simulink model "Ultrafiltration"  (R2025b)
settings: Solver=FixedStepAuto  StartTime=0.0  StopTime=1440  FixedStep=1  RelTol=1e-3
InitFcn:
  | initUF
  | tic;
StartFcn:
  | disp("Start...")
StopFcn:
  | disp("Stop...")
  | fprintf("SimTime: %.02f min", toc/60)
values from neighbouring files (symbols this model uses):
  BW_Max_Time = 90    [initUF.m]
  BW_Max_Vol_gal = 5000    [initUF.m]
  CEB_Max_Time = 1000    [initUF.m]
  CEB_Max_Vol_gal = 5000    [initUF.m]
  CIP_Max_Time = 15000    [initUF.m]
undefined symbols (not defined in the file or in its folder): LUT
libraries: simulink x30
(part 1 of 5)
PostSaveFcn:
  | disp("PostSave...")
PauseFcn:
  | disp("Pause...")
settings Model: Creator=joshl  LastModifiedBy=joshl
settings RTWCC: GPUComputeCapability=3.5

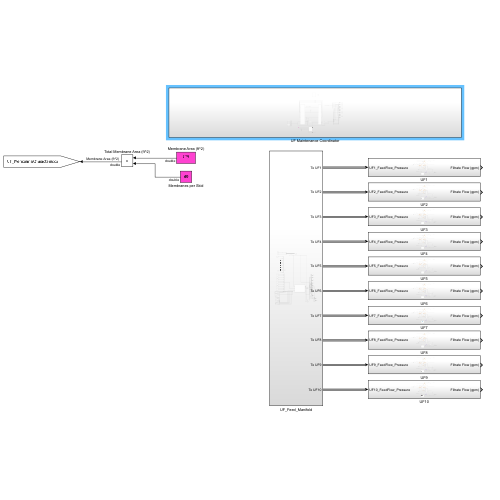
[thumbnail: Simulink's stored preview of the top-level diagram]
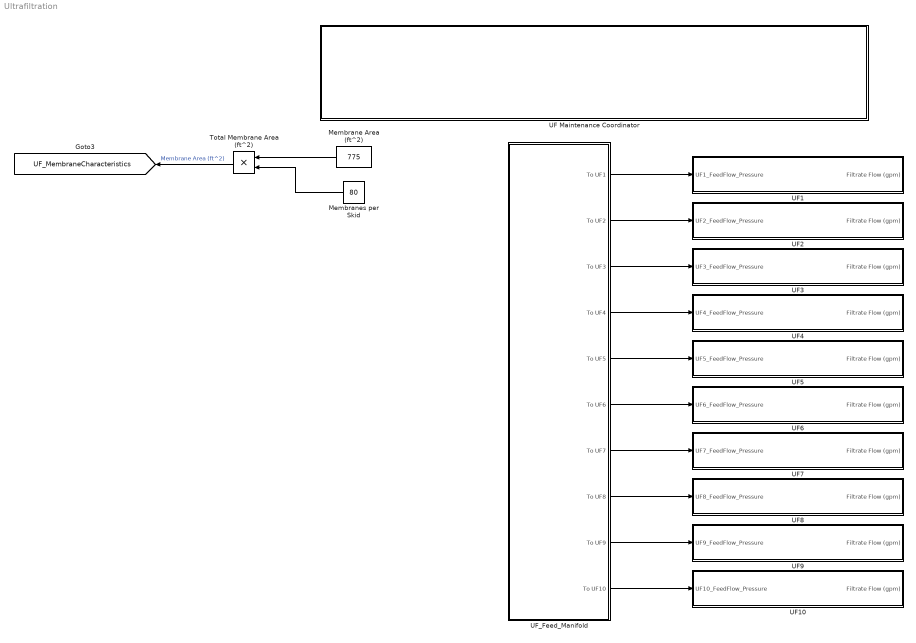
== system Ultrafiltration ==
  Membrane Area (ft^2) : Constant  Value=775
  Membranes per Skid : Constant  Value=80
  Total Membrane Area (ft^2) : Product
  UF Maintenance Coordinator : Subsystem
  UF1 : Subsystem
  UF10 : Subsystem
  UF2 : Subsystem
  UF3 : Subsystem
  UF4 : Subsystem
  UF5 : Subsystem
  UF6 : Subsystem
  UF7 : Subsystem
  UF8 : Subsystem
  UF9 : Subsystem
  UF_Feed_Manifold : Subsystem
  tag scope: UF_MembraneCharacteristics=global
  wires:
  UF_Feed_Manifold/1(To UF1) -> UF1/1(UF1_FeedFlow_Pressure)
  UF_Feed_Manifold/2(To UF2) -> UF2/1(UF2_FeedFlow_Pressure)
  Membrane Area (ft^2)/1 -> Total Membrane Area (ft^2)/1
  Membranes per Skid/1 -> Total Membrane Area (ft^2)/2
  Total Membrane Area (ft^2)/1 -> [UF_MembraneCharacteristics]  "Membrane Area (ft^2)"
  UF_Feed_Manifold/3(To UF3) -> UF3/1(UF3_FeedFlow_Pressure)
  UF_Feed_Manifold/4(To UF4) -> UF4/1(UF4_FeedFlow_Pressure)
  UF_Feed_Manifold/5(To UF5) -> UF5/1(UF5_FeedFlow_Pressure)
  UF_Feed_Manifold/6(To UF6) -> UF6/1(UF6_FeedFlow_Pressure)
  UF_Feed_Manifold/7(To UF7) -> UF7/1(UF7_FeedFlow_Pressure)
  UF_Feed_Manifold/8(To UF8) -> UF8/1(UF8_FeedFlow_Pressure)
  UF_Feed_Manifold/9(To UF9) -> UF9/1(UF9_FeedFlow_Pressure)
  UF_Feed_Manifold/10(To UF10) -> UF10/1(UF10_FeedFlow_Pressure)

== system Ultrafiltration/UF Maintenance Coordinator ==
  Bus Creator{,1..9} (10 alike) : BusCreator  Inputs=2
  Constant : Constant  Value=10000
  Demux : Demux  Outputs=10
  Demux1 : Demux  Outputs=10
  Maint Queue Vector2 : Mux  Inputs=10
  Memory{,1..3} (4 alike) : Memory
  Rate Limiter : RateLimiter  RisingSlewLimit=10000/108  FallingSlewLimit=-10000/37  SampleTimeMode=inherited
  Sample_Stateflows : Stateflow chart  Commented=on  TreatAsAtomicUnit=on
  Scope : Scope  NumInputPorts=2
      settings: DataLoggingVariableName=ScopeData2
  Scope1 : Scope  NumInputPorts=3
      settings: ActiveDisplayYMinimum=-0.12499999999999997  ActiveDisplayYMaximum=1.125
  Scope{2..5} (4 alike) : Scope
      Scope2 settings: ActiveDisplayYMinimum=-1  ActiveDisplayYMaximum=1  DataLoggingVariableName=ScopeData14
      Scope3 settings: ActiveDisplayYMinimum=-1  ActiveDisplayYMaximum=1  DataLoggingVariableName=ScopeData15
      Scope4 settings: ActiveDisplayYMinimum=-129.2228584451866  ActiveDisplayYMaximum=1163.0057260066797  DataLoggingVariableName=ScopeData16
      Scope5 settings: ActiveDisplayYMinimum=-1.2345292012789748  ActiveDisplayYMaximum=1.3904707987210259  DataLoggingVariableName=ScopeData17
  Scope6 : Scope  NumInputPorts=2
      settings: ActiveDisplayYMinimum=-0.12499999999999997  ActiveDisplayYMaximum=1.125  DataLoggingVariableName=ScopeData18
  UF Flow Maximum (gpm) : Constant  Value=1640
  UF_Dispatcher : MATLAB Function  TreatAsAtomicUnit=on
  UF_FIFO_Coordinator : MATLAB Function  Priority=100  TreatAsAtomicUnit=on  SystemSampleTime=1
  UF_State_Tracker : MATLAB Function  TreatAsAtomicUnit=on  SystemSampleTime=1
  arhive : Subsystem
  tag scope: UF10_State=global, UF1_State=global, UF2_State=global, UF3_State=global, UF4_State=global, UF5_State=global, UF6_State=global, UF7_State=global, UF8_State=global, UF9_State=global, UF_Flow_Assignment=global, UF_Operations_States_vector=global
  wires:
  UF_State_Tracker/3(operations_states) -> Scope5/1, [UF_Operations_States_vector], UF_FIFO_Coordinator/3(operating_states)
  UF_State_Tracker/1(in_startup_queue) -> Scope3/1, UF_FIFO_Coordinator/1(startup_req)
  UF_State_Tracker/2(in_maint_queue) -> Scope2/1, UF_FIFO_Coordinator/2(maint_req)
  UF_State_Tracker/4(maintenance_completion_indicators) -> Scope6/1, Scope1/3, [UF_Maintenance_Completion_Signals]  "Maintenance Completion"
  UF_FIFO_Coordinator/1(startup_cmd) -> Memory/1
  UF_FIFO_Coordinator/2(maint_cmd) -> Memory1/1
  Memory/1 -> UF_State_Tracker/1(startup_cmd)
  Memory1/1 -> UF_State_Tracker/2(maint_cmd)
  UF_FIFO_Coordinator/3(shutdown_cmd) -> Memory2/1
  Memory2/1 -> UF_State_Tracker/3(shutdown_cmd)
  UF_Dispatcher/1(flows) -> UF_FIFO_Coordinator/4(flows), Scope4/1, Memory3/1
  Rate Limiter/1 -> Scope/1, UF_Dispatcher/2(flow_actual)  "Plant Feed Actual"
  Memory3/1 -> UF_Dispatcher/4(prev_flows)
  UF Flow Maximum (gpm)/1 -> UF_Dispatcher/1(max_flow_per_unit)
  [UF2_Maintenance_Request] -> Maint Queue Vector2/2
  [UF3_Maintenance_Request] -> Maint Queue Vector2/3
  [UF7_Maintenance_Request] -> Maint Queue Vector2/7
  [UF8_Maintenance_Request] -> Maint Queue Vector2/8
  [UF5_Maintenance_Request] -> Maint Queue Vector2/5
  [UF6_Maintenance_Request] -> Maint Queue Vector2/6
  [UF10_Maintenance_Request] -> Maint Queue Vector2/10
  [UF9_Maintenance_Request] -> Maint Queue Vector2/9
  [UF4_Maintenance_Request] -> Maint Queue Vector2/4
  [UF1_Maintenance_Request] -> Maint Queue Vector2/1
  [UF_Maintenance_Completion_Signals] -> Demux/1
  Maint Queue Vector2/1 -> Scope6/2, UF_State_Tracker/4(maint_req)
  Constant/1 -> Rate Limiter/1, Scope/2, UF_Dispatcher/3(flow_setpoint)
  Demux/1 -> Bus Creator/1  "UF1_MaintenanceCompletion_signal"
  Bus Creator/1 -> [UF1_State]
  Demux/2 -> Bus Creator1/1  "UF2_MaintenanceCompletion_signal"
  Demux/3 -> Bus Creator2/1  "UF3_MaintenanceCompletion_signal"
  Demux/4 -> Bus Creator3/1  "UF4_MaintenanceCompletion_signal"
  Demux/5 -> Bus Creator4/1  "UF5_MaintenanceCompletion_signal"
  Bus Creator1/1 -> [UF2_State]
  Demux/6 -> Bus Creator5/1  "UF6_MaintenanceCompletion_signal"
  Bus Creator3/1 -> [UF4_State]
  Bus Creator2/1 -> [UF3_State]
  Bus Creator5/1 -> [UF6_State]
  Bus Creator4/1 -> [UF5_State]
  Bus Creator7/1 -> [UF8_State]
  Bus Creator6/1 -> [UF7_State]
  Bus Creator9/1 -> [UF10_State]
  Bus Creator8/1 -> [UF9_State]
  Demux/7 -> Bus Creator6/1  "UF7_MaintenanceCompletion_signal"
  Demux/8 -> Bus Creator7/1  "UF8_MaintenanceCompletion_signal"
  Demux/9 -> Bus Creator8/1  "UF9_MaintenanceCompletion_signal"
  Demux/10 -> Bus Creator9/1  "UF10_MaintenanceCompletion_signal"
  Demux1/2 -> Bus Creator1/2  "UF2_OperationsState_signal"
  Demux1/7 -> Bus Creator6/2  "UF7_OperationsState_signal"
  Demux1/10 -> Bus Creator9/2  "UF10_OperationsState_signal"
  Demux1/1 -> Bus Creator/2  "UF1_OperationsState_signal"
  Demux1/8 -> Bus Creator7/2  "UF8_OperationsState_signal"
  Demux1/4 -> Bus Creator3/2  "UF4_OperationsState_signal"
  Demux1/9 -> Bus Creator8/2  "UF9_OperationsState_signal"
  Demux1/3 -> Bus Creator2/2  "UF3_OperationsState_signal"
  [UF_Operations_States_vector] -> Scope1/1, Demux1/1  "OperationsStates"
  Demux1/5 -> Bus Creator4/2  "UF5_OperationsState_signal"
  Demux1/6 -> Bus Creator5/2  "UF6_OperationsState_signal"
  UF_FIFO_Coordinator/4(assigned_flows) -> Scope1/2, [UF_Flow_Assignment]  "Flows"

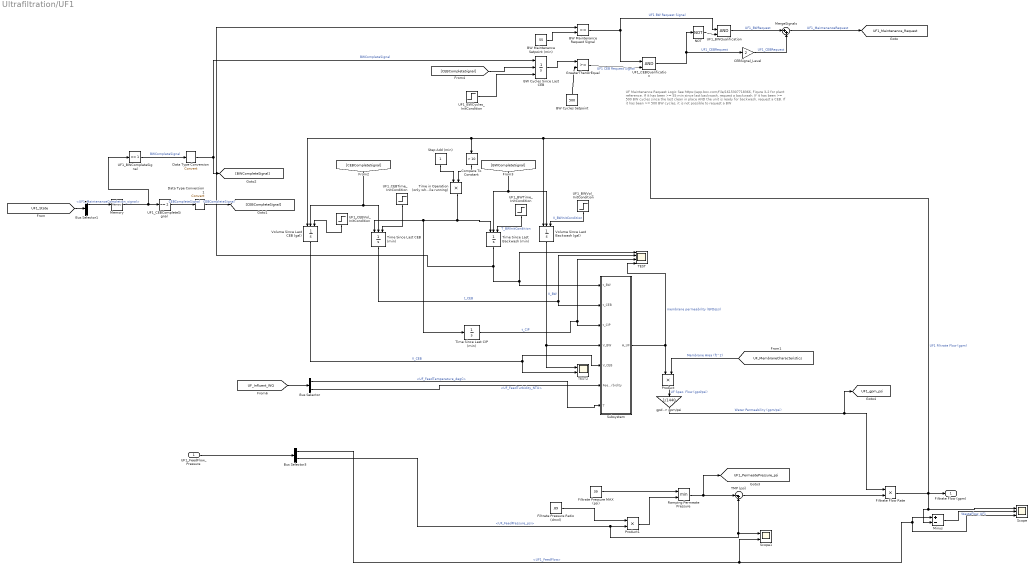
== system Ultrafiltration/UF1 ==
  note: UF Maintenance Request Logic
      | See https://app.box.com/file/1615307718366, Figure 3-2 for plant reference.
      |
      | If it has been >= 55 min since last backwash, request a backwash.
      | If it has been >= 500 BW cycles since the last clean in place AND the unit is ready for backwash, request a CEB.
      | If it has been >= 500 BW cycles, it is not possible to request a BW
  UF1_FeedFlow_Pressure : Inport
  BW Cycles Setpoint : Constant  Value=500
  BW Cycles Since Last CEB : Integrator  ExternalReset=rising  InitialConditionSource=external  InitialCondition=5
  BW Maintenance Request Signal : RelationalOperator  OutDataTypeStr=boolean  RndMeth=Simplest  InputSameDT=off
  BW Maintenance Setpoint (min) : Constant  Value=55
  Bus Selector : BusSelector  OutputSignals=UF_FeedTemperature_degC,UF_FeedTurbidity_NTU
  Bus Selector1 : BusSelector  OutputSignals=UF1_MaintenanceCompletion_signal,UF1_OperationsState_signal
  Bus Selector3 : BusSelector  OutputSignals=UF1_FeedFlow,UF_FeedPressure_psi
  CEBSignal_Level : Gain  Gain=2  OutDataTypeStr=double
  Compare To Constant : simulink/Logic and Bit Operations/Compare To Constant  relop=>  const=10  OutDataTypeStr=boolean
  Data Type Conversion : DataTypeConversion  SaturateOnIntegerOverflow=off  RndMeth=Floor
  Data Type Conversion1 : DataTypeConversion  SaturateOnIntegerOverflow=off  RndMeth=Floor
  Filtrate Flow Rate : Product
  Filtrate Pressure MAX (psi) : Constant  Value=39
  Filtrate Pressure Ratio (dmnl) : Constant  Value=.89
  GreaterThanOrEqual : RelationalOperator  OutDataTypeStr=boolean  RndMeth=Simplest  InputSameDT=off
  Memory : Memory
  MergeSignals : Sum  Inputs=|++
  Minus : Sum  Inputs=+-
  NOT : Logic  Operator=NOT  IconShape=distinctive  AllPortsSameDT=off  OutDataTypeStr=boolean
  Product : Product
  Product1 : Product
  Ramping Permeate Pressure : MinMax  Inputs=2
  Scope : Scope  NumInputPorts=3
      settings: ActiveDisplayYMinimum=-126.71796384165732  ActiveDisplayYMaximum=1140.4616745749161  DataLoggingVariableName=ScopeData10
  Scope1 : Scope  NumInputPorts=2
      settings: ActiveDisplayYMinimum=-178.57142857142856  ActiveDisplayYMaximum=1607.1428571428573  DataLoggingVariableName=ScopeData11
  Step Add (min) : Constant
  Subsystem : Subsystem
  TEST : Scope  NumInputPorts=4
      settings: ActiveDisplayYMinimum=13.625  ActiveDisplayYMaximum=27.375  DataLoggingVariableName=ScopeData3
  TEST2 : Scope  NumInputPorts=2
      settings: ActiveDisplayYMinimum=-311929.86683332996  ActiveDisplayYMaximum=2.8073688014999703E+6  DataLoggingVariableName=ScopeData4
  TMP (psi) : Sum  Inputs=|-+
  Time Since Last Backwash (min) : Integrator  ExternalReset=level hold  InitialConditionSource=external  InitialCondition=26
  Time Since Last CEB (min) : Integrator  ExternalReset=level hold  InitialConditionSource=external  InitialCondition=4833
  Time Since Last CIP (min) : Integrator  InitialCondition=round(CIP_Max_Time*rand())
  Time in Operation (only while running) : Product
  UF1_BWCompleteSignal : simulink/Logic and Bit Operations/Compare To Constant  relop===  const=1  OutDataTypeStr=uint8
  UF1_BWCycles_InitCondition : Step  Before=round(500 * rand())  After=0  SampleTime=0
  UF1_BWQualification : Logic  IconShape=distinctive  AllPortsSameDT=off  OutDataTypeStr=boolean
  UF1_BWTime_InitCondition : Step  Before=round(BW_Max_Time*rand())  After=0  SampleTime=0
  UF1_BWVol_InitCondition : Step  Before=round(BW_Max_Vol_gal*rand())  After=0  SampleTime=0
  UF1_CEBCompleteSignal : simulink/Logic and Bit Operations/Compare To Constant  relop===  const=2  OutDataTypeStr=uint8
  UF1_CEBQualification : Logic  IconShape=distinctive  AllPortsSameDT=off  OutDataTypeStr=boolean
  UF1_CEBTime_InitCondition : Step  Before=round(CEB_Max_Time*rand())  After=0  SampleTime=0
  UF1_CEBVol_InitCondition : Step  Before=round(CEB_Max_Vol_gal*rand())  After=0  SampleTime=0
  Volume Since Last Backwash (gal) : Integrator  ExternalReset=level hold  InitialConditionSource=external  InitialCondition=34330
  Volume Since Last CEB (gal) : Integrator  ExternalReset=rising  InitialConditionSource=external  InitialCondition=2777254
  "gpd -> gpm/psi" : Gain  Gain=1/1440
  Filtrate Flow (gpm) : Outport
  tag scope: UF1_Maintenance_Request=global, UF1_PermeatePressure_psi=global, UF1_gpm_psi=global
  wires:
  Volume Since Last Backwash (gal)/1 -> Subsystem/4(V_BW), TEST2/1  "V_BW"
  Time Since Last Backwash (min)/1 -> BW Maintenance Request Signal/1, Subsystem/1(t_BW), TEST/1
  Product/1 -> "gpd -> gpm/psi"/1  "UF Spec. Flow (gpd/psi)"
  [UF_MembraneCharacteristics] -> Product/2  "Membrane Area (ft^2)"
  "gpd -> gpm/psi"/1 -> Filtrate Flow Rate/1, [UF1_gpm_psi]  "Water Permeability (gpm/psi)"
  Time in Operation (only while running)/1 -> Time Since Last Backwash (min)/1, Time Since Last CEB (min)/1, Time Since Last CIP (min)/1
  Filtrate Flow Rate/1 -> Scope/1, Minus/2, Volume Since Last Backwash (gal)/1, Volume Since Last CEB (gal)/1, Compare To Constant/1, Filtrate Flow (gpm)/1  "UF1 Filtrate Flow (gpm)"
  Time Since Last CEB (min)/1 -> Subsystem/2(t_CEB), TEST/2  "t_CEB"
  Volume Since Last CEB (gal)/1 -> Subsystem/5(V_CEB), TEST2/2  "V_CEB"
  Time Since Last CIP (min)/1 -> Subsystem/3(t_CIP), TEST/3  "t_CIP"
  Filtrate Pressure MAX (psi)/1 -> Ramping Permeate Pressure/1
  [UF_Influent_WQ] -> Bus Selector/1
  Bus Selector/1 -> Subsystem/7(T)  "<UF_FeedTemperature_degC>"
  UF1_FeedFlow_Pressure/1 -> Bus Selector3/1
  Filtrate Pressure Ratio (dmnl)/1 -> Product1/1
  Product1/1 -> Ramping Permeate Pressure/2
  Ramping Permeate Pressure/1 -> [UF1_PermeatePressure_psi], TMP (psi)/1
  TMP (psi)/1 -> Filtrate Flow Rate/2
  BW Maintenance Setpoint (min)/1 -> BW Maintenance Request Signal/2
  BW Cycles Since Last CEB/1 -> GreaterThanOrEqual/1
  BW Cycles Setpoint/1 -> GreaterThanOrEqual/2
  Bus Selector/2 -> Subsystem/6(Feed Turbidity)  "<UF_FeedTurbidity_NTU>"
  [UF1_State] -> Bus Selector1/1
  MergeSignals/1 -> [UF1_Maintenance_Request]  "UF1_MaintenanceRequest"
  UF1_CEBCompleteSignal/1 -> Data Type Conversion1/1  "CEBCompleteSignal"
  [CEBCompleteSignal] -> Volume Since Last CEB (gal)/2, Time Since Last CEB (min)/2
  Data Type Conversion/1 -> [BWCompleteSignal], BW Cycles Since Last CEB/1  "BWCompleteSignal"
  [BWCompleteSignal] -> Volume Since Last Backwash (gal)/2, Time Since Last Backwash (min)/2
  [CEBCompleteSignal] -> BW Cycles Since Last CEB/2
  Bus Selector1/1 -> Memory/1  "<UF1_MaintenanceCompletion_signal>"
  UF1_BWCompleteSignal/1 -> Data Type Conversion/1  "BWCompleteSignal"
  Data Type Conversion1/1 -> [CEBCompleteSignal]  "CEBCompleteSignal"
  UF1_BWCycles_InitCondition/1 -> BW Cycles Since Last CEB/3
  Subsystem/1(A_UF) -> TEST/4, Product/1  "membrane permeability (GFD/psi)"
  UF1_BWTime_InitCondition/1 -> Time Since Last Backwash (min)/3  "T_BWInitCondition"
  UF1_CEBVol_InitCondition/1 -> Volume Since Last CEB (gal)/3
  UF1_CEBTime_InitCondition/1 -> Time Since Last CEB (min)/3
  UF1_BWVol_InitCondition/1 -> Volume Since Last Backwash (gal)/3  "V_BWInitCondition"
  Step Add (min)/1 -> Time in Operation (only while running)/1
  Compare To Constant/1 -> Time in Operation (only while running)/2
  Memory/1 -> UF1_BWCompleteSignal/1, UF1_CEBCompleteSignal/1
  UF1_BWQualification/1 -> MergeSignals/1  "UF1_BWRequest"
  GreaterThanOrEqual/1 -> UF1_CEBQualification/2  "UF1 CEB Request Signal"
  UF1_CEBQualification/1 -> CEBSignal_Level/1, NOT/1  "UF1_CEBRequest"
  BW Maintenance Request Signal/1 -> UF1_BWQualification/1, UF1_CEBQualification/1  "UF1 BW Request Signal"
  NOT/1 -> UF1_BWQualification/2
  CEBSignal_Level/1 -> MergeSignals/2  "UF1_CEBRequest"
  Bus Selector3/1 -> Scope1/2, Minus/1, Scope/3  "<UF1_FeedFlow>"
  Bus Selector3/2 -> TMP (psi)/2, Scope1/1, Product1/2  "<UF_FeedPressure_psi>"
  Minus/1 -> Scope/2  "WasteFlow_UF1"

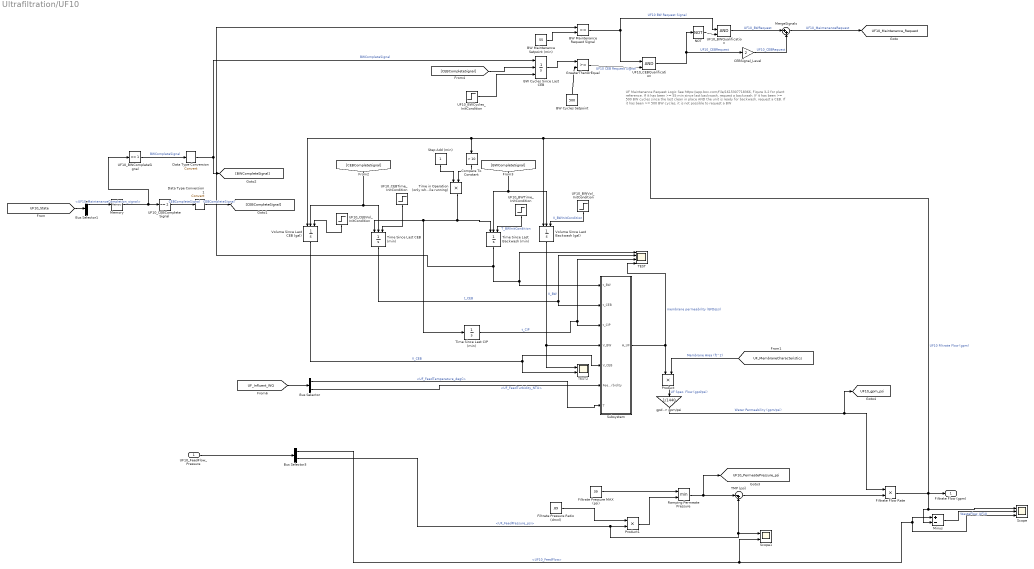
== system Ultrafiltration/UF10 ==
  note: UF Maintenance Request Logic
      | See https://app.box.com/file/1615307718366, Figure 3-2 for plant reference.
      |
      | If it has been >= 55 min since last backwash, request a backwash.
      | If it has been >= 500 BW cycles since the last clean in place AND the unit is ready for backwash, request a CEB.
      | If it has been >= 500 BW cycles, it is not possible to request a BW
  UF10_FeedFlow_Pressure : Inport
  BW Cycles Setpoint : Constant  Value=500
  BW Cycles Since Last CEB : Integrator  ExternalReset=rising  InitialConditionSource=external  InitialCondition=5
  BW Maintenance Request Signal : RelationalOperator  OutDataTypeStr=boolean  RndMeth=Simplest  InputSameDT=off
  BW Maintenance Setpoint (min) : Constant  Value=55
  Bus Selector : BusSelector  OutputSignals=UF_FeedTemperature_degC,UF_FeedTurbidity_NTU
  Bus Selector1 : BusSelector  OutputSignals=UF10_MaintenanceCompletion_signal,UF10_OperationsState_signal
  Bus Selector3 : BusSelector  OutputSignals=UF10_FeedFlow,UF_FeedPressure_psi
  CEBSignal_Level : Gain  Gain=2  OutDataTypeStr=double
  Compare To Constant : simulink/Logic and Bit Operations/Compare To Constant  relop=>  const=10  OutDataTypeStr=boolean
  Data Type Conversion : DataTypeConversion  SaturateOnIntegerOverflow=off  RndMeth=Floor
  Data Type Conversion1 : DataTypeConversion  SaturateOnIntegerOverflow=off  RndMeth=Floor
  Filtrate Flow Rate : Product
  Filtrate Pressure MAX (psi) : Constant  Value=39
  Filtrate Pressure Ratio (dmnl) : Constant  Value=.89
  GreaterThanOrEqual : RelationalOperator  OutDataTypeStr=boolean  RndMeth=Simplest  InputSameDT=off
  Memory : Memory
  MergeSignals : Sum  Inputs=|++
  Minus : Sum  Inputs=+-
  NOT : Logic  Operator=NOT  IconShape=distinctive  AllPortsSameDT=off  OutDataTypeStr=boolean
  Product : Product
  Product1 : Product
  Ramping Permeate Pressure : MinMax  Inputs=2
  Scope : Scope  NumInputPorts=3
      settings: ActiveDisplayYMinimum=-126.71796384165732  ActiveDisplayYMaximum=1140.4616745749161  DataLoggingVariableName=ScopeData10
  Scope1 : Scope  NumInputPorts=2
      settings: ActiveDisplayYMinimum=-129.2228584451866  ActiveDisplayYMaximum=1163.0057260066797  DataLoggingVariableName=ScopeData11
  Step Add (min) : Constant
  Subsystem : Subsystem
  TEST : Scope  NumInputPorts=4
      settings: ActiveDisplayYMinimum=13.625  ActiveDisplayYMaximum=27.375  DataLoggingVariableName=ScopeData3
  TEST2 : Scope  NumInputPorts=2
      settings: ActiveDisplayYMinimum=-311929.86683332996  ActiveDisplayYMaximum=2.8073688014999703E+6  DataLoggingVariableName=ScopeData4
  TMP (psi) : Sum  Inputs=|-+
  Time Since Last Backwash (min) : Integrator  ExternalReset=level hold  InitialConditionSource=external  InitialCondition=26
  Time Since Last CEB (min) : Integrator  ExternalReset=level hold  InitialConditionSource=external  InitialCondition=4833
  Time Since Last CIP (min) : Integrator  InitialCondition=round(CIP_Max_Time*rand())
  Time in Operation (only while running) : Product
  UF10_BWCompleteSignal : simulink/Logic and Bit Operations/Compare To Constant  relop===  const=1  OutDataTypeStr=uint8
  UF10_BWCycles_InitCondition : Step  Before=round(500 * rand())  After=0  SampleTime=0
  UF10_BWQualification : Logic  IconShape=distinctive  AllPortsSameDT=off  OutDataTypeStr=boolean
  UF10_BWTime_InitCondition : Step  Before=round(BW_Max_Time*rand())  After=0  SampleTime=0
  UF10_BWVol_InitCondition : Step  Before=round(BW_Max_Vol_gal*rand())  After=0  SampleTime=0
  UF10_CEBCompleteSignal : simulink/Logic and Bit Operations/Compare To Constant  relop===  const=2  OutDataTypeStr=uint8
  UF10_CEBQualification : Logic  IconShape=distinctive  AllPortsSameDT=off  OutDataTypeStr=boolean
  UF10_CEBTime_InitCondition : Step  Before=round(CEB_Max_Time*rand())  After=0  SampleTime=0
  UF10_CEBVol_InitCondition : Step  Before=round(CEB_Max_Vol_gal*rand())  After=0  SampleTime=0
  Volume Since Last Backwash (gal) : Integrator  ExternalReset=level hold  InitialConditionSource=external  InitialCondition=34330
  Volume Since Last CEB (gal) : Integrator  ExternalReset=rising  InitialConditionSource=external  InitialCondition=2777254
  "gpd -> gpm/psi" : Gain  Gain=1/1440
  Filtrate Flow (gpm) : Outport
  tag scope: UF10_Maintenance_Request=global, UF10_PermeatePressure_psi=global, UF10_gpm_psi=global
  wires:
  Volume Since Last Backwash (gal)/1 -> Subsystem/4(V_BW), TEST2/1  "V_BW"
  Time Since Last Backwash (min)/1 -> BW Maintenance Request Signal/1, Subsystem/1(t_BW), TEST/1
  Product/1 -> "gpd -> gpm/psi"/1  "UF Spec. Flow (gpd/psi)"
  [UF_MembraneCharacteristics] -> Product/2  "Membrane Area (ft^2)"
  "gpd -> gpm/psi"/1 -> Filtrate Flow Rate/1, [UF10_gpm_psi]  "Water Permeability (gpm/psi)"
  Time in Operation (only while running)/1 -> Time Since Last Backwash (min)/1, Time Since Last CEB (min)/1, Time Since Last CIP (min)/1
  Filtrate Flow Rate/1 -> Scope/1, Minus/2, Volume Since Last Backwash (gal)/1, Volume Since Last CEB (gal)/1, Compare To Constant/1, Filtrate Flow (gpm)/1  "UF10 Filtrate Flow (gpm)"
  Time Since Last CEB (min)/1 -> Subsystem/2(t_CEB), TEST/2  "t_CEB"
  Volume Since Last CEB (gal)/1 -> Subsystem/5(V_CEB), TEST2/2  "V_CEB"
  Time Since Last CIP (min)/1 -> Subsystem/3(t_CIP), TEST/3  "t_CIP"
  Filtrate Pressure MAX (psi)/1 -> Ramping Permeate Pressure/1
  [UF_Influent_WQ] -> Bus Selector/1
  Bus Selector/1 -> Subsystem/7(T)  "<UF_FeedTemperature_degC>"
  UF10_FeedFlow_Pressure/1 -> Bus Selector3/1
  Filtrate Pressure Ratio (dmnl)/1 -> Product1/1
  Product1/1 -> Ramping Permeate Pressure/2
  Ramping Permeate Pressure/1 -> [UF10_PermeatePressure_psi], TMP (psi)/1
  TMP (psi)/1 -> Filtrate Flow Rate/2
  BW Maintenance Setpoint (min)/1 -> BW Maintenance Request Signal/2
  BW Cycles Since Last CEB/1 -> GreaterThanOrEqual/1
  BW Cycles Setpoint/1 -> GreaterThanOrEqual/2
  Bus Selector/2 -> Subsystem/6(Feed Turbidity)  "<UF_FeedTurbidity_NTU>"
  [UF10_State] -> Bus Selector1/1
  MergeSignals/1 -> [UF10_Maintenance_Request]  "UF10_MaintenanceRequest"
  UF10_CEBCompleteSignal/1 -> Data Type Conversion1/1  "CEBCompleteSignal"
  [CEBCompleteSignal] -> Volume Since Last CEB (gal)/2, Time Since Last CEB (min)/2
  Data Type Conversion/1 -> [BWCompleteSignal], BW Cycles Since Last CEB/1  "BWCompleteSignal"
  [BWCompleteSignal] -> Volume Since Last Backwash (gal)/2, Time Since Last Backwash (min)/2
  [CEBCompleteSignal] -> BW Cycles Since Last CEB/2
  Bus Selector1/1 -> Memory/1  "<UF10_MaintenanceCompletion_signal>"
  UF10_BWCompleteSignal/1 -> Data Type Conversion/1  "BWCompleteSignal"
  Data Type Conversion1/1 -> [CEBCompleteSignal]  "CEBCompleteSignal"
  UF10_BWCycles_InitCondition/1 -> BW Cycles Since Last CEB/3
  Subsystem/1(A_UF) -> TEST/4, Product/1  "membrane permeability (GFD/psi)"
  UF10_BWTime_InitCondition/1 -> Time Since Last Backwash (min)/3  "T_BWInitCondition"
  UF10_CEBVol_InitCondition/1 -> Volume Since Last CEB (gal)/3
  UF10_CEBTime_InitCondition/1 -> Time Since Last CEB (min)/3
  UF10_BWVol_InitCondition/1 -> Volume Since Last Backwash (gal)/3  "V_BWInitCondition"
  Step Add (min)/1 -> Time in Operation (only while running)/1
  Compare To Constant/1 -> Time in Operation (only while running)/2
  Memory/1 -> UF10_BWCompleteSignal/1, UF10_CEBCompleteSignal/1
  UF10_BWQualification/1 -> MergeSignals/1  "UF10_BWRequest"
  GreaterThanOrEqual/1 -> UF10_CEBQualification/2  "UF10 CEB Request Signal"
  UF10_CEBQualification/1 -> CEBSignal_Level/1, NOT/1  "UF10_CEBRequest"
  BW Maintenance Request Signal/1 -> UF10_BWQualification/1, UF10_CEBQualification/1  "UF10 BW Request Signal"
  NOT/1 -> UF10_BWQualification/2
  CEBSignal_Level/1 -> MergeSignals/2  "UF10_CEBRequest"
  Bus Selector3/1 -> Scope1/2, Minus/1, Scope/3  "<UF10_FeedFlow>"
  Bus Selector3/2 -> TMP (psi)/2, Scope1/1, Product1/2  "<UF_FeedPressure_psi>"
  Minus/1 -> Scope/2  "WasteFlow_UF10"

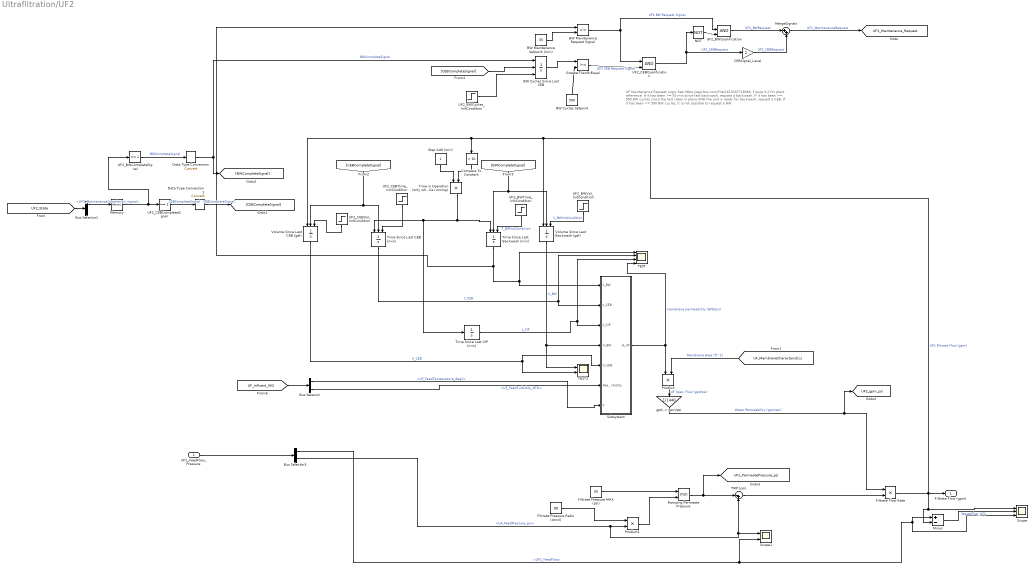
== system Ultrafiltration/UF2 ==
  note: UF Maintenance Request Logic
      | See https://app.box.com/file/1615307718366, Figure 3-2 for plant reference.
      |
      | If it has been >= 55 min since last backwash, request a backwash.
      | If it has been >= 500 BW cycles since the last clean in place AND the unit is ready for backwash, request a CEB.
      | If it has been >= 500 BW cycles, it is not possible to request a BW
  UF2_FeedFlow_Pressure : Inport
  BW Cycles Setpoint : Constant  Value=500
  BW Cycles Since Last CEB : Integrator  ExternalReset=rising  InitialConditionSource=external  InitialCondition=5
  BW Maintenance Request Signal : RelationalOperator  OutDataTypeStr=boolean  RndMeth=Simplest  InputSameDT=off
  BW Maintenance Setpoint (min) : Constant  Value=55
  Bus Selector : BusSelector  OutputSignals=UF_FeedTemperature_degC,UF_FeedTurbidity_NTU
  Bus Selector1 : BusSelector  OutputSignals=UF2_MaintenanceCompletion_signal,UF2_OperationsState_signal
  Bus Selector3 : BusSelector  OutputSignals=UF2_FeedFlow,UF_FeedPressure_psi
  CEBSignal_Level : Gain  Gain=2  OutDataTypeStr=double
  Compare To Constant : simulink/Logic and Bit Operations/Compare To Constant  relop=>  const=10  OutDataTypeStr=boolean
  Data Type Conversion : DataTypeConversion  SaturateOnIntegerOverflow=off  RndMeth=Floor
  Data Type Conversion1 : DataTypeConversion  SaturateOnIntegerOverflow=off  RndMeth=Floor
  Filtrate Flow Rate : Product
  Filtrate Pressure MAX (psi) : Constant  Value=39
  Filtrate Pressure Ratio (dmnl) : Constant  Value=.89
  GreaterThanOrEqual : RelationalOperator  OutDataTypeStr=boolean  RndMeth=Simplest  InputSameDT=off
  Memory : Memory
  MergeSignals : Sum  Inputs=|++
  Minus : Sum  Inputs=+-
  NOT : Logic  Operator=NOT  IconShape=distinctive  AllPortsSameDT=off  OutDataTypeStr=boolean
  Product : Product
  Product1 : Product
  Ramping Permeate Pressure : MinMax  Inputs=2
  Scope : Scope  NumInputPorts=3
      settings: ActiveDisplayYMinimum=-126.71796384165732  ActiveDisplayYMaximum=1140.4616745749161  DataLoggingVariableName=ScopeData10
  Scope1 : Scope  NumInputPorts=2
      settings: ActiveDisplayYMinimum=-129.2228584451866  ActiveDisplayYMaximum=1163.0057260066797  DataLoggingVariableName=ScopeData11
  Step Add (min) : Constant
  Subsystem : Subsystem
  TEST : Scope  NumInputPorts=4
      settings: ActiveDisplayYMinimum=13.625  ActiveDisplayYMaximum=27.375  DataLoggingVariableName=ScopeData3
  TEST2 : Scope  NumInputPorts=2
      settings: ActiveDisplayYMinimum=-311929.86683332996  ActiveDisplayYMaximum=2.8073688014999703E+6  DataLoggingVariableName=ScopeData4
  TMP (psi) : Sum  Inputs=|-+
  Time Since Last Backwash (min) : Integrator  ExternalReset=level hold  InitialConditionSource=external  InitialCondition=26
  Time Since Last CEB (min) : Integrator  ExternalReset=level hold  InitialConditionSource=external  InitialCondition=4833
  Time Since Last CIP (min) : Integrator  InitialCondition=round(CIP_Max_Time*rand())
  Time in Operation (only while running) : Product
  UF2_BWCompleteSignal : simulink/Logic and Bit Operations/Compare To Constant  relop===  const=1  OutDataTypeStr=uint8
  UF2_BWCycles_InitCondition : Step  Before=round(500 * rand())  After=0  SampleTime=0
  UF2_BWQualification : Logic  IconShape=distinctive  AllPortsSameDT=off  OutDataTypeStr=boolean
  UF2_BWTime_InitCondition : Step  Before=round(BW_Max_Time*rand())  After=0  SampleTime=0
  UF2_BWVol_InitCondition : Step  Before=round(BW_Max_Vol_gal*rand())  After=0  SampleTime=0
  UF2_CEBCompleteSignal : simulink/Logic and Bit Operations/Compare To Constant  relop===  const=2  OutDataTypeStr=uint8
  UF2_CEBQualification : Logic  IconShape=distinctive  AllPortsSameDT=off  OutDataTypeStr=boolean
  UF2_CEBTime_InitCondition : Step  Before=round(CEB_Max_Time*rand())  After=0  SampleTime=0
  UF2_CEBVol_InitCondition : Step  Before=round(CEB_Max_Vol_gal*rand())  After=0  SampleTime=0
  Volume Since Last Backwash (gal) : Integrator  ExternalReset=level hold  InitialConditionSource=external  InitialCondition=34330
  Volume Since Last CEB (gal) : Integrator  ExternalReset=rising  InitialConditionSource=external  InitialCondition=2777254
  "gpd -> gpm/psi" : Gain  Gain=1/1440
  Filtrate Flow (gpm) : Outport
  tag scope: UF2_Maintenance_Request=global, UF2_PermeatePressure_psi=global, UF2_gpm_psi=global
  wires:
  Volume Since Last Backwash (gal)/1 -> Subsystem/4(V_BW), TEST2/1  "V_BW"
  Time Since Last Backwash (min)/1 -> BW Maintenance Request Signal/1, Subsystem/1(t_BW), TEST/1
  Product/1 -> "gpd -> gpm/psi"/1  "UF Spec. Flow (gpd/psi)"
  [UF_MembraneCharacteristics] -> Product/2  "Membrane Area (ft^2)"
  "gpd -> gpm/psi"/1 -> Filtrate Flow Rate/1, [UF2_gpm_psi]  "Water Permeability (gpm/psi)"
  Time in Operation (only while running)/1 -> Time Since Last Backwash (min)/1, Time Since Last CEB (min)/1, Time Since Last CIP (min)/1
  Filtrate Flow Rate/1 -> Scope/1, Minus/2, Volume Since Last Backwash (gal)/1, Volume Since Last CEB (gal)/1, Compare To Constant/1, Filtrate Flow (gpm)/1  "UF2 Filtrate Flow (gpm)"
  Time Since Last CEB (min)/1 -> Subsystem/2(t_CEB), TEST/2  "t_CEB"
  Volume Since Last CEB (gal)/1 -> Subsystem/5(V_CEB), TEST2/2  "V_CEB"
  Time Since Last CIP (min)/1 -> Subsystem/3(t_CIP), TEST/3  "t_CIP"
  Filtrate Pressure MAX (psi)/1 -> Ramping Permeate Pressure/1
  [UF_Influent_WQ] -> Bus Selector/1
  Bus Selector/1 -> Subsystem/7(T)  "<UF_FeedTemperature_degC>"
  UF2_FeedFlow_Pressure/1 -> Bus Selector3/1
  Filtrate Pressure Ratio (dmnl)/1 -> Product1/1
  Product1/1 -> Ramping Permeate Pressure/2
  Ramping Permeate Pressure/1 -> [UF2_PermeatePressure_psi], TMP (psi)/1
  TMP (psi)/1 -> Filtrate Flow Rate/2
  BW Maintenance Setpoint (min)/1 -> BW Maintenance Request Signal/2
  BW Cycles Since Last CEB/1 -> GreaterThanOrEqual/1
  BW Cycles Setpoint/1 -> GreaterThanOrEqual/2
  Bus Selector/2 -> Subsystem/6(Feed Turbidity)  "<UF_FeedTurbidity_NTU>"
  [UF2_State] -> Bus Selector1/1
  MergeSignals/1 -> [UF2_Maintenance_Request]  "UF2_MaintenanceRequest"
  UF2_CEBCompleteSignal/1 -> Data Type Conversion1/1  "CEBCompleteSignal"
  [CEBCompleteSignal] -> Volume Since Last CEB (gal)/2, Time Since Last CEB (min)/2
  Data Type Conversion/1 -> [BWCompleteSignal], BW Cycles Since Last CEB/1  "BWCompleteSignal"
  [BWCompleteSignal] -> Volume Since Last Backwash (gal)/2, Time Since Last Backwash (min)/2
  [CEBCompleteSignal] -> BW Cycles Since Last CEB/2
  Bus Selector1/1 -> Memory/1  "<UF2_MaintenanceCompletion_signal>"
  UF2_BWCompleteSignal/1 -> Data Type Conversion/1  "BWCompleteSignal"
  Data Type Conversion1/1 -> [CEBCompleteSignal]  "CEBCompleteSignal"
  UF2_BWCycles_InitCondition/1 -> BW Cycles Since Last CEB/3
  Subsystem/1(A_UF) -> TEST/4, Product/1  "membrane permeability (GFD/psi)"
  UF2_BWTime_InitCondition/1 -> Time Since Last Backwash (min)/3  "T_BWInitCondition"
  UF2_CEBVol_InitCondition/1 -> Volume Since Last CEB (gal)/3
  UF2_CEBTime_InitCondition/1 -> Time Since Last CEB (min)/3
  UF2_BWVol_InitCondition/1 -> Volume Since Last Backwash (gal)/3  "V_BWInitCondition"
  Step Add (min)/1 -> Time in Operation (only while running)/1
  Compare To Constant/1 -> Time in Operation (only while running)/2
  Memory/1 -> UF2_BWCompleteSignal/1, UF2_CEBCompleteSignal/1
  UF2_BWQualification/1 -> MergeSignals/1  "UF2_BWRequest"
  GreaterThanOrEqual/1 -> UF2_CEBQualification/2  "UF2 CEB Request Signal"
  UF2_CEBQualification/1 -> CEBSignal_Level/1, NOT/1  "UF2_CEBRequest"
  BW Maintenance Request Signal/1 -> UF2_BWQualification/1, UF2_CEBQualification/1  "UF2 BW Request Signal"
  NOT/1 -> UF2_BWQualification/2
  CEBSignal_Level/1 -> MergeSignals/2  "UF2_CEBRequest"
  Bus Selector3/1 -> Scope1/2, Minus/1, Scope/3  "<UF2_FeedFlow>"
  Bus Selector3/2 -> TMP (psi)/2, Scope1/1, Product1/2  "<UF_FeedPressure_psi>"
  Minus/1 -> Scope/2  "WasteFlow_UF2"

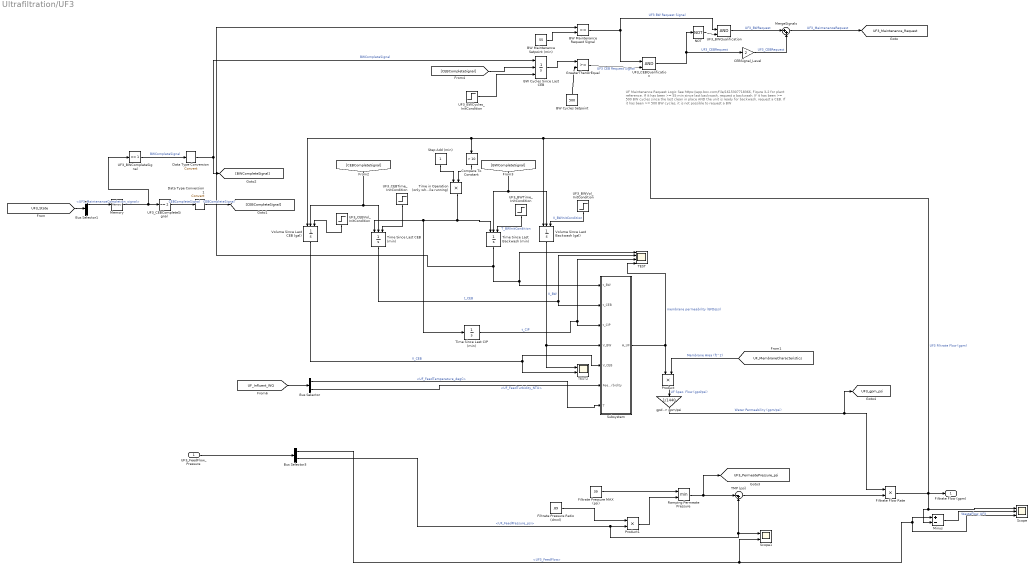
== system Ultrafiltration/UF3 ==
  note: UF Maintenance Request Logic
      | See https://app.box.com/file/1615307718366, Figure 3-2 for plant reference.
      |
      | If it has been >= 55 min since last backwash, request a backwash.
      | If it has been >= 500 BW cycles since the last clean in place AND the unit is ready for backwash, request a CEB.
      | If it has been >= 500 BW cycles, it is not possible to request a BW
  UF3_FeedFlow_Pressure : Inport
  BW Cycles Setpoint : Constant  Value=500
  BW Cycles Since Last CEB : Integrator  ExternalReset=rising  InitialConditionSource=external  InitialCondition=5
  BW Maintenance Request Signal : RelationalOperator  OutDataTypeStr=boolean  RndMeth=Simplest  InputSameDT=off
  BW Maintenance Setpoint (min) : Constant  Value=55
  Bus Selector : BusSelector  OutputSignals=UF_FeedTemperature_degC,UF_FeedTurbidity_NTU
  Bus Selector1 : BusSelector  OutputSignals=UF3_MaintenanceCompletion_signal,UF3_OperationsState_signal
  Bus Selector3 : BusSelector  OutputSignals=UF3_FeedFlow,UF_FeedPressure_psi
  CEBSignal_Level : Gain  Gain=2  OutDataTypeStr=double
  Compare To Constant : simulink/Logic and Bit Operations/Compare To Constant  relop=>  const=10  OutDataTypeStr=boolean
  Data Type Conversion : DataTypeConversion  SaturateOnIntegerOverflow=off  RndMeth=Floor
  Data Type Conversion1 : DataTypeConversion  SaturateOnIntegerOverflow=off  RndMeth=Floor
  Filtrate Flow Rate : Product
  Filtrate Pressure MAX (psi) : Constant  Value=39
  Filtrate Pressure Ratio (dmnl) : Constant  Value=.89
  GreaterThanOrEqual : RelationalOperator  OutDataTypeStr=boolean  RndMeth=Simplest  InputSameDT=off
  Memory : Memory
  MergeSignals : Sum  Inputs=|++
  Minus : Sum  Inputs=+-
  NOT : Logic  Operator=NOT  IconShape=distinctive  AllPortsSameDT=off  OutDataTypeStr=boolean
  Product : Product
  Product1 : Product
  Ramping Permeate Pressure : MinMax  Inputs=2
  Scope : Scope  NumInputPorts=3
      settings: ActiveDisplayYMinimum=-126.71796384165732  ActiveDisplayYMaximum=1140.4616745749161  DataLoggingVariableName=ScopeData10
  Scope1 : Scope  NumInputPorts=2
      settings: ActiveDisplayYMinimum=-129.2228584451866  ActiveDisplayYMaximum=1163.0057260066797  DataLoggingVariableName=ScopeData11
  Step Add (min) : Constant
  Subsystem : Subsystem
  TEST : Scope  NumInputPorts=4
      settings: ActiveDisplayYMinimum=13.625  ActiveDisplayYMaximum=27.375  DataLoggingVariableName=ScopeData3
  TEST2 : Scope  NumInputPorts=2
      settings: ActiveDisplayYMinimum=-311929.86683332996  ActiveDisplayYMaximum=2.8073688014999703E+6  DataLoggingVariableName=ScopeData4
  TMP (psi) : Sum  Inputs=|-+
  Time Since Last Backwash (min) : Integrator  ExternalReset=level hold  InitialConditionSource=external  InitialCondition=26
  Time Since Last CEB (min) : Integrator  ExternalReset=level hold  InitialConditionSource=external  InitialCondition=4833
  Time Since Last CIP (min) : Integrator  InitialCondition=round(CIP_Max_Time*rand())
  Time in Operation (only while running) : Product
  UF3_BWCompleteSignal : simulink/Logic and Bit Operations/Compare To Constant  relop===  const=1  OutDataTypeStr=uint8
  UF3_BWCycles_InitCondition : Step  Before=round(500 * rand())  After=0  SampleTime=0
  UF3_BWQualification : Logic  IconShape=distinctive  AllPortsSameDT=off  OutDataTypeStr=boolean
  UF3_BWTime_InitCondition : Step  Before=round(BW_Max_Time*rand())  After=0  SampleTime=0
  UF3_BWVol_InitCondition : Step  Before=round(BW_Max_Vol_gal*rand())  After=0  SampleTime=0
  UF3_CEBCompleteSignal : simulink/Logic and Bit Operations/Compare To Constant  relop===  const=2  OutDataTypeStr=uint8
  UF3_CEBQualification : Logic  IconShape=distinctive  AllPortsSameDT=off  OutDataTypeStr=boolean
  UF3_CEBTime_InitCondition : Step  Before=round(CEB_Max_Time*rand())  After=0  SampleTime=0
  UF3_CEBVol_InitCondition : Step  Before=round(CEB_Max_Vol_gal*rand())  After=0  SampleTime=0
  Volume Since Last Backwash (gal) : Integrator  ExternalReset=level hold  InitialConditionSource=external  InitialCondition=34330
  Volume Since Last CEB (gal) : Integrator  ExternalReset=rising  InitialConditionSource=external  InitialCondition=2777254
  "gpd -> gpm/psi" : Gain  Gain=1/1440
  Filtrate Flow (gpm) : Outport
  tag scope: UF3_Maintenance_Request=global, UF3_PermeatePressure_psi=global, UF3_gpm_psi=global
  wires:
  Volume Since Last Backwash (gal)/1 -> Subsystem/4(V_BW), TEST2/1  "V_BW"
  Time Since Last Backwash (min)/1 -> BW Maintenance Request Signal/1, Subsystem/1(t_BW), TEST/1
  Product/1 -> "gpd -> gpm/psi"/1  "UF Spec. Flow (gpd/psi)"
  [UF_MembraneCharacteristics] -> Product/2  "Membrane Area (ft^2)"
  "gpd -> gpm/psi"/1 -> Filtrate Flow Rate/1, [UF3_gpm_psi]  "Water Permeability (gpm/psi)"
  Time in Operation (only while running)/1 -> Time Since Last Backwash (min)/1, Time Since Last CEB (min)/1, Time Since Last CIP (min)/1
  Filtrate Flow Rate/1 -> Scope/1, Minus/2, Volume Since Last Backwash (gal)/1, Volume Since Last CEB (gal)/1, Compare To Constant/1, Filtrate Flow (gpm)/1  "UF3 Filtrate Flow (gpm)"
  Time Since Last CEB (min)/1 -> Subsystem/2(t_CEB), TEST/2  "t_CEB"
  Volume Since Last CEB (gal)/1 -> Subsystem/5(V_CEB), TEST2/2  "V_CEB"
  Time Since Last CIP (min)/1 -> Subsystem/3(t_CIP), TEST/3  "t_CIP"
  Filtrate Pressure MAX (psi)/1 -> Ramping Permeate Pressure/1
  [UF_Influent_WQ] -> Bus Selector/1
  Bus Selector/1 -> Subsystem/7(T)  "<UF_FeedTemperature_degC>"
  UF3_FeedFlow_Pressure/1 -> Bus Selector3/1
  Filtrate Pressure Ratio (dmnl)/1 -> Product1/1
  Product1/1 -> Ramping Permeate Pressure/2
  Ramping Permeate Pressure/1 -> [UF3_PermeatePressure_psi], TMP (psi)/1
  TMP (psi)/1 -> Filtrate Flow Rate/2
  BW Maintenance Setpoint (min)/1 -> BW Maintenance Request Signal/2
  BW Cycles Since Last CEB/1 -> GreaterThanOrEqual/1
  BW Cycles Setpoint/1 -> GreaterThanOrEqual/2
  Bus Selector/2 -> Subsystem/6(Feed Turbidity)  "<UF_FeedTurbidity_NTU>"
  [UF3_State] -> Bus Selector1/1
  MergeSignals/1 -> [UF3_Maintenance_Request]  "UF3_MaintenanceRequest"
  UF3_CEBCompleteSignal/1 -> Data Type Conversion1/1  "CEBCompleteSignal"
  [CEBCompleteSignal] -> Volume Since Last CEB (gal)/2, Time Since Last CEB (min)/2
  Data Type Conversion/1 -> [BWCompleteSignal], BW Cycles Since Last CEB/1  "BWCompleteSignal"
  [BWCompleteSignal] -> Volume Since Last Backwash (gal)/2, Time Since Last Backwash (min)/2
  [CEBCompleteSignal] -> BW Cycles Since Last CEB/2
  Bus Selector1/1 -> Memory/1  "<UF3_MaintenanceCompletion_signal>"
  UF3_BWCompleteSignal/1 -> Data Type Conversion/1  "BWCompleteSignal"
  Data Type Conversion1/1 -> [CEBCompleteSignal]  "CEBCompleteSignal"
  UF3_BWCycles_InitCondition/1 -> BW Cycles Since Last CEB/3
  Subsystem/1(A_UF) -> TEST/4, Product/1  "membrane permeability (GFD/psi)"
  UF3_BWTime_InitCondition/1 -> Time Since Last Backwash (min)/3  "T_BWInitCondition"
  UF3_CEBVol_InitCondition/1 -> Volume Since Last CEB (gal)/3
  UF3_CEBTime_InitCondition/1 -> Time Since Last CEB (min)/3
  UF3_BWVol_InitCondition/1 -> Volume Since Last Backwash (gal)/3  "V_BWInitCondition"
  Step Add (min)/1 -> Time in Operation (only while running)/1
  Compare To Constant/1 -> Time in Operation (only while running)/2
  Memory/1 -> UF3_BWCompleteSignal/1, UF3_CEBCompleteSignal/1
  UF3_BWQualification/1 -> MergeSignals/1  "UF3_BWRequest"
  GreaterThanOrEqual/1 -> UF3_CEBQualification/2  "UF3 CEB Request Signal"
  UF3_CEBQualification/1 -> CEBSignal_Level/1, NOT/1  "UF3_CEBRequest"
  BW Maintenance Request Signal/1 -> UF3_BWQualification/1, UF3_CEBQualification/1  "UF3 BW Request Signal"
  NOT/1 -> UF3_BWQualification/2
  CEBSignal_Level/1 -> MergeSignals/2  "UF3_CEBRequest"
  Bus Selector3/1 -> Scope1/2, Minus/1, Scope/3  "<UF3_FeedFlow>"
  Bus Selector3/2 -> TMP (psi)/2, Scope1/1, Product1/2  "<UF_FeedPressure_psi>"
  Minus/1 -> Scope/2  "WasteFlow_UF3"

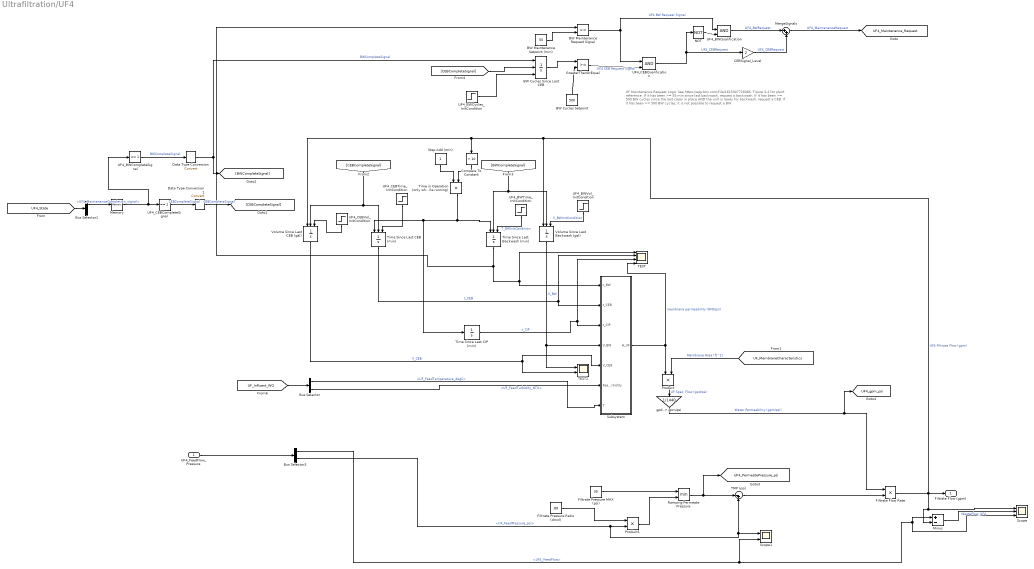
== system Ultrafiltration/UF4 ==
  note: UF Maintenance Request Logic
      | See https://app.box.com/file/1615307718366, Figure 3-2 for plant reference.
      |
      | If it has been >= 55 min since last backwash, request a backwash.
      | If it has been >= 500 BW cycles since the last clean in place AND the unit is ready for backwash, request a CEB.
      | If it has been >= 500 BW cycles, it is not possible to request a BW
  UF4_FeedFlow_Pressure : Inport
  BW Cycles Setpoint : Constant  Value=500
  BW Cycles Since Last CEB : Integrator  ExternalReset=rising  InitialConditionSource=external  InitialCondition=5
  BW Maintenance Request Signal : RelationalOperator  OutDataTypeStr=boolean  RndMeth=Simplest  InputSameDT=off
  BW Maintenance Setpoint (min) : Constant  Value=55
  Bus Selector : BusSelector  OutputSignals=UF_FeedTemperature_degC,UF_FeedTurbidity_NTU
  Bus Selector1 : BusSelector  OutputSignals=UF4_MaintenanceCompletion_signal,UF4_OperationsState_signal
  Bus Selector3 : BusSelector  OutputSignals=UF4_FeedFlow,UF_FeedPressure_psi
  CEBSignal_Level : Gain  Gain=2  OutDataTypeStr=double
  Compare To Constant : simulink/Logic and Bit Operations/Compare To Constant  relop=>  const=10  OutDataTypeStr=boolean
  Data Type Conversion : DataTypeConversion  SaturateOnIntegerOverflow=off  RndMeth=Floor
  Data Type Conversion1 : DataTypeConversion  SaturateOnIntegerOverflow=off  RndMeth=Floor
  Filtrate Flow Rate : Product
  Filtrate Pressure MAX (psi) : Constant  Value=39
  Filtrate Pressure Ratio (dmnl) : Constant  Value=.89
  GreaterThanOrEqual : RelationalOperator  OutDataTypeStr=boolean  RndMeth=Simplest  InputSameDT=off
  Memory : Memory
  MergeSignals : Sum  Inputs=|++
  Minus : Sum  Inputs=+-
  NOT : Logic  Operator=NOT  IconShape=distinctive  AllPortsSameDT=off  OutDataTypeStr=boolean
  Product : Product
  Product1 : Product
  Ramping Permeate Pressure : MinMax  Inputs=2
  Scope : Scope  NumInputPorts=3
      settings: ActiveDisplayYMinimum=-126.71796384165732  ActiveDisplayYMaximum=1140.4616745749161  DataLoggingVariableName=ScopeData10
  Scope1 : Scope  NumInputPorts=2
      settings: ActiveDisplayYMinimum=-129.2228584451866  ActiveDisplayYMaximum=1163.0057260066797  DataLoggingVariableName=ScopeData11
  Step Add (min) : Constant
  Subsystem : Subsystem
  TEST : Scope  NumInputPorts=4
      settings: ActiveDisplayYMinimum=13.625  ActiveDisplayYMaximum=27.375  DataLoggingVariableName=ScopeData3
  TEST2 : Scope  NumInputPorts=2
      settings: ActiveDisplayYMinimum=-311929.86683332996  ActiveDisplayYMaximum=2.8073688014999703E+6  DataLoggingVariableName=ScopeData4
  TMP (psi) : Sum  Inputs=|-+
  Time Since Last Backwash (min) : Integrator  ExternalReset=level hold  InitialConditionSource=external  InitialCondition=26
  Time Since Last CEB (min) : Integrator  ExternalReset=level hold  InitialConditionSource=external  InitialCondition=4833
  Time Since Last CIP (min) : Integrator  InitialCondition=round(CIP_Max_Time*rand())
  Time in Operation (only while running) : Product
  UF4_BWCompleteSignal : simulink/Logic and Bit Operations/Compare To Constant  relop===  const=1  OutDataTypeStr=uint8
  UF4_BWCycles_InitCondition : Step  Before=round(500 * rand())  After=0  SampleTime=0
  UF4_BWQualification : Logic  IconShape=distinctive  AllPortsSameDT=off  OutDataTypeStr=boolean
  UF4_BWTime_InitCondition : Step  Before=round(BW_Max_Time*rand())  After=0  SampleTime=0
  UF4_BWVol_InitCondition : Step  Before=round(BW_Max_Vol_gal*rand())  After=0  SampleTime=0
  UF4_CEBCompleteSignal : simulink/Logic and Bit Operations/Compare To Constant  relop===  const=2  OutDataTypeStr=uint8
  UF4_CEBQualification : Logic  IconShape=distinctive  AllPortsSameDT=off  OutDataTypeStr=boolean
  UF4_CEBTime_InitCondition : Step  Before=round(CEB_Max_Time*rand())  After=0  SampleTime=0
  UF4_CEBVol_InitCondition : Step  Before=round(CEB_Max_Vol_gal*rand())  After=0  SampleTime=0
  Volume Since Last Backwash (gal) : Integrator  ExternalReset=level hold  InitialConditionSource=external  InitialCondition=34330
  Volume Since Last CEB (gal) : Integrator  ExternalReset=rising  InitialConditionSource=external  InitialCondition=2777254
  "gpd -> gpm/psi" : Gain  Gain=1/1440
  Filtrate Flow (gpm) : Outport
  tag scope: UF4_Maintenance_Request=global, UF4_PermeatePressure_psi=global, UF4_gpm_psi=global
  wires:
  Volume Since Last Backwash (gal)/1 -> Subsystem/4(V_BW), TEST2/1  "V_BW"
  Time Since Last Backwash (min)/1 -> BW Maintenance Request Signal/1, Subsystem/1(t_BW), TEST/1
  Product/1 -> "gpd -> gpm/psi"/1  "UF Spec. Flow (gpd/psi)"
  [UF_MembraneCharacteristics] -> Product/2  "Membrane Area (ft^2)"
  "gpd -> gpm/psi"/1 -> Filtrate Flow Rate/1, [UF4_gpm_psi]  "Water Permeability (gpm/psi)"
  Time in Operation (only while running)/1 -> Time Since Last Backwash (min)/1, Time Since Last CEB (min)/1, Time Since Last CIP (min)/1
  Filtrate Flow Rate/1 -> Scope/1, Minus/2, Volume Since Last Backwash (gal)/1, Volume Since Last CEB (gal)/1, Compare To Constant/1, Filtrate Flow (gpm)/1  "UF4 Filtrate Flow (gpm)"
  Time Since Last CEB (min)/1 -> Subsystem/2(t_CEB), TEST/2  "t_CEB"
  Volume Since Last CEB (gal)/1 -> Subsystem/5(V_CEB), TEST2/2  "V_CEB"
  Time Since Last CIP (min)/1 -> Subsystem/3(t_CIP), TEST/3  "t_CIP"
  Filtrate Pressure MAX (psi)/1 -> Ramping Permeate Pressure/1
  [UF_Influent_WQ] -> Bus Selector/1
  Bus Selector/1 -> Subsystem/7(T)  "<UF_FeedTemperature_degC>"
  UF4_FeedFlow_Pressure/1 -> Bus Selector3/1
  Filtrate Pressure Ratio (dmnl)/1 -> Product1/1
  Product1/1 -> Ramping Permeate Pressure/2
  Ramping Permeate Pressure/1 -> [UF4_PermeatePressure_psi], TMP (psi)/1
  TMP (psi)/1 -> Filtrate Flow Rate/2
  BW Maintenance Setpoint (min)/1 -> BW Maintenance Request Signal/2
  BW Cycles Since Last CEB/1 -> GreaterThanOrEqual/1
  BW Cycles Setpoint/1 -> GreaterThanOrEqual/2
  Bus Selector/2 -> Subsystem/6(Feed Turbidity)  "<UF_FeedTurbidity_NTU>"
  [UF4_State] -> Bus Selector1/1
  MergeSignals/1 -> [UF4_Maintenance_Request]  "UF4_MaintenanceRequest"
  UF4_CEBCompleteSignal/1 -> Data Type Conversion1/1  "CEBCompleteSignal"
  [CEBCompleteSignal] -> Volume Since Last CEB (gal)/2, Time Since Last CEB (min)/2
  Data Type Conversion/1 -> [BWCompleteSignal], BW Cycles Since Last CEB/1  "BWCompleteSignal"
  [BWCompleteSignal] -> Volume Since Last Backwash (gal)/2, Time Since Last Backwash (min)/2
  [CEBCompleteSignal] -> BW Cycles Since Last CEB/2
  Bus Selector1/1 -> Memory/1  "<UF4_MaintenanceCompletion_signal>"
  UF4_BWCompleteSignal/1 -> Data Type Conversion/1  "BWCompleteSignal"
  Data Type Conversion1/1 -> [CEBCompleteSignal]  "CEBCompleteSignal"
  UF4_BWCycles_InitCondition/1 -> BW Cycles Since Last CEB/3
  Subsystem/1(A_UF) -> TEST/4, Product/1  "membrane permeability (GFD/psi)"
  UF4_BWTime_InitCondition/1 -> Time Since Last Backwash (min)/3  "T_BWInitCondition"
  UF4_CEBVol_InitCondition/1 -> Volume Since Last CEB (gal)/3
  UF4_CEBTime_InitCondition/1 -> Time Since Last CEB (min)/3
  UF4_BWVol_InitCondition/1 -> Volume Since Last Backwash (gal)/3  "V_BWInitCondition"
  Step Add (min)/1 -> Time in Operation (only while running)/1
  Compare To Constant/1 -> Time in Operation (only while running)/2
  Memory/1 -> UF4_BWCompleteSignal/1, UF4_CEBCompleteSignal/1
  UF4_BWQualification/1 -> MergeSignals/1  "UF4_BWRequest"
  GreaterThanOrEqual/1 -> UF4_CEBQualification/2  "UF4 CEB Request Signal"
  UF4_CEBQualification/1 -> CEBSignal_Level/1, NOT/1  "UF4_CEBRequest"
  BW Maintenance Request Signal/1 -> UF4_BWQualification/1, UF4_CEBQualification/1  "UF4 BW Request Signal"
  NOT/1 -> UF4_BWQualification/2
  CEBSignal_Level/1 -> MergeSignals/2  "UF4_CEBRequest"
  Bus Selector3/1 -> Scope1/2, Minus/1, Scope/3  "<UF4_FeedFlow>"
  Bus Selector3/2 -> TMP (psi)/2, Scope1/1, Product1/2  "<UF_FeedPressure_psi>"
  Minus/1 -> Scope/2  "WasteFlow_UF4"
